simulink model "smm_gait_control"  (R2018b)
settings: configuration reference "Configuration1khz" (kept outside this file)
InitFcn:
  | addpath('./functions/')
  | addpath('./policies/')
  | control_params
values from neighbouring files (symbols this model uses):
  rest = extract_policy_variables('policies/rest.mat')    [control_params.m]
  run_slow = extract_policy_variables('policies/06_run_reduced.mat')    [control_params.m]
  walk_slow = extract_policy_variables('policies/06_walk.mat')    [control_params.m]
undefined symbols (not defined in the file or in its folder): ctrl, Discrete, initial_dx_estimate, initial_dy_estimate, initial_dz_estimate, initial_z_estimate, sample_time, Time
libraries: simulink x42, ctrlSharedLib x7
(part 1 of 5)
settings Model: Creator=wmartin  LastModifiedBy=Will
settings ConfigSetRef: SourceLocation=Base Workspace

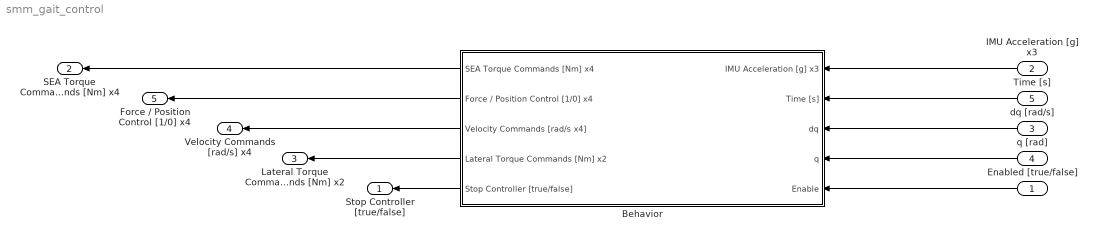
== system smm_gait_control ==
  Enabled [true/false] : Inport  OutDataTypeStr=boolean  PortDimensions=1  SampleTime=sample_time  Interpolate=off
  IMU Acceleration [g] x3 : Inport  Port=2  OutDataTypeStr=double  PortDimensions=3  SampleTime=sample_time  Interpolate=off
  dq [rad/s] : Inport  Port=3  OutDataTypeStr=double  PortDimensions=13  SampleTime=sample_time  Interpolate=off
  q [rad] : Inport  Port=4  OutDataTypeStr=double  PortDimensions=13  SampleTime=sample_time  Interpolate=off
  Time [s] : Inport  Port=5  OutDataTypeStr=double  PortDimensions=1  SampleTime=sample_time  Interpolate=off
  Behavior : Subsystem
  Stop Controller [true/false] : Outport  OutDataTypeStr=boolean  PortDimensions=1  SampleTime=[0.001,0]  OutputWhenDisabled=reset  InitialOutput=[0 0 0 0 0 0]
  SEA Torque Commands [Nm] x4 : Outport  Port=2  OutDataTypeStr=double  PortDimensions=4  SampleTime=[0.001,0]  OutputWhenDisabled=reset  InitialOutput=[0 0 0 0 0 0]
  Lateral Torque Commands [Nm] x2 : Outport  Port=3  OutDataTypeStr=double  PortDimensions=2  SampleTime=[0.001,0]  OutputWhenDisabled=reset  InitialOutput=[0 0 0 0 0 0]
  Velocity Commands [rad/s] x4 : Outport  Port=4  OutDataTypeStr=double  PortDimensions=4  SampleTime=[0.001,0]  OutputWhenDisabled=reset  InitialOutput=[0 0 0 0 0 0]
  Force / Position Control [1/0] x4 : Outport  Port=5  OutDataTypeStr=boolean  PortDimensions=4  SampleTime=[0.001,0]  OutputWhenDisabled=reset  InitialOutput=[0 0 0 0 0 0]
  wires:
  IMU Acceleration [g] x3/1 -> Behavior/1(IMU Acceleration [g] x3)
  dq [rad/s]/1 -> Behavior/3(dq)
  q [rad]/1 -> Behavior/4(q)
  Time [s]/1 -> Behavior/2(Time [s])
  Enabled [true/false]/1 -> Behavior/5(Enable)
  Behavior/5(Stop Controller [true/false]) -> Stop Controller [true/false]/1
  Behavior/1(SEA Torque Commands [Nm] x4) -> SEA Torque Commands [Nm] x4/1
  Behavior/2(Force / Position Control [1/0] x4) -> Force / Position Control [1/0] x4/1
  Behavior/3(Velocity Commands [rad/s x4]) -> Velocity Commands [rad/s] x4/1
  Behavior/4(Lateral Torque Commands [Nm] x2) -> Lateral Torque Commands [Nm] x2/1

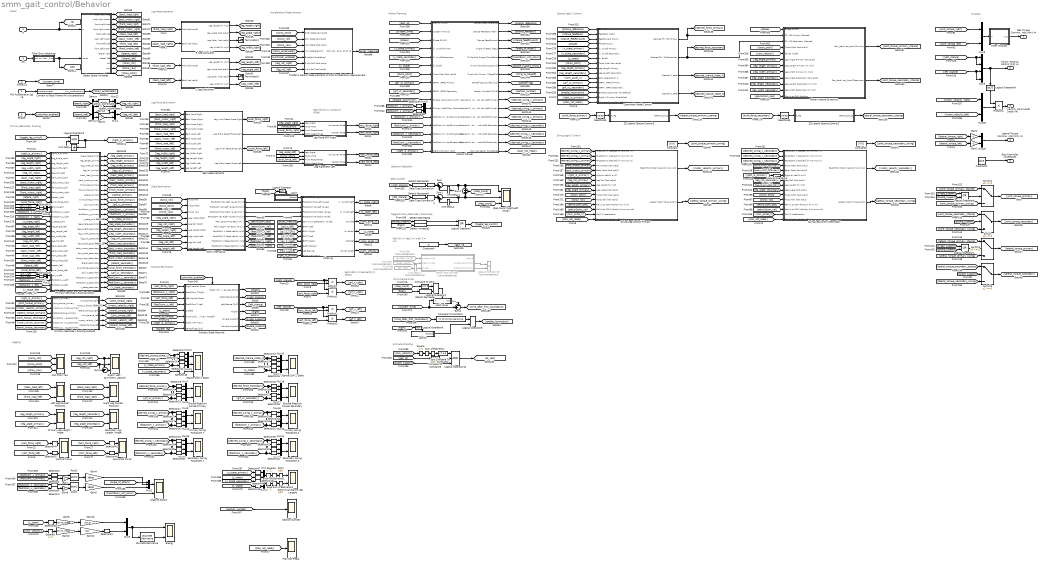
== system smm_gait_control/Behavior ==
  note: Step counter
  note: Gait ID
      | 1 = rest
      | 2 = walk
      | 3 = run
  note: Each GRF is 2 elements
      | [F, dF/dt]
  note: Primary/Secondary Routing
  note: Leg Measurements
  note: Outputs
  note: Inputs
  note: Contact Estimation
  note: Logging
  note: Acceleration Measurement
  note: Swing Leg(s) Control
  note: Leg Force Estimation
  note: Each force is 2 values
      | [F, dF/dt]
  note: State Estimation
  note: Behavior Selection
  note: Toggle Primary/Secondary Role Swap
  note: First stance timer
  note: Activate standing
  note: Motion Planning
  note: Stance Leg(s) Control
  IMU Acceleration [g] x3 : Inport  OutDataTypeStr=double  PortDimensions=3  SampleTime=[0.001,0]
  Time [s] : Inport  Port=2  OutDataTypeStr=double  PortDimensions=1  SampleTime=[0.001,0]
  dq : Inport  Port=3  OutDataTypeStr=double  PortDimensions=13  SampleTime=[0.001,0]
  q : Inport  Port=4  OutDataTypeStr=double  PortDimensions=13  SampleTime=[0.001,0]
  Enable : Inport  Port=5  OutDataTypeStr=boolean  PortDimensions=1  SampleTime=[0.001,0]
  2D Lateral Stance Control2 : MATLAB Function  TreatAsAtomicUnit=on
  2D Lateral Stance Control3 : MATLAB Function  TreatAsAtomicUnit=on
  Angle of Attack : Scope  NumInputPorts=2
  Atan1 : Trigonometry  Operator=atan2
  Atan2 : Trigonometry  Operator=atan2
  Centroidal Model Control : Subsystem
  CoM Kinematics : Subsystem
  Compare To Constant : simulink/Logic and Bit Operations/Compare To Constant  relop=>=  const=ctrl.control_start_time  OutDataTypeStr=boolean
  Compare To Constant2 : simulink/Logic and Bit Operations/Compare To Constant  relop=<=  const=0.5  OutDataTypeStr=boolean
  Compare To Constant3 : simulink/Logic and Bit Operations/Compare To Constant  relop===  const=1  OutDataTypeStr=boolean
  Compare To Zero : simulink/Logic and Bit Operations/Compare To Zero  relop===  OutDataTypeStr=boolean
  Constant : Constant  Value=[0 0]
  Constant2 : Constant  Value=false
  Constant4 : Constant  Value=3
  Constant5 : Constant  Value=[0 0]
  Contact State Machine : Subsystem
  Convert to Body Frame IMU Accelerations : MATLAB Function  TreatAsAtomicUnit=on
  Data Type Conversion : DataTypeConversion  OutDataTypeStr=double
  Data Type Conversion1 : DataTypeConversion  OutDataTypeStr=double
  Demux : Demux  Outputs=2
  Demux1 : Demux  Outputs=2
  Detect Decrease : simulink/Logic and Bit Operations/Detect Decrease  vinit=0.0  OutDataTypeStr=boolean
  Detect Decrease2 : simulink/Logic and Bit Operations/Detect Decrease  vinit=0  OutDataTypeStr=boolean
  Detect Decrease3 : simulink/Logic and Bit Operations/Detect Decrease  vinit=0.0  OutDataTypeStr=boolean
  Detect Decrease4 : simulink/Logic and Bit Operations/Detect Decrease  vinit=0  OutDataTypeStr=boolean
  Detect Increase2 : simulink/Logic and Bit Operations/Detect Increase  vinit=1  OutDataTypeStr=boolean
  Discrete Derivative : simulink/Discrete/Discrete Derivative  gainval=1.0  ICPrevScaledInput=0.0  OutMin=[]  OutMax=[]  OutDataType=fixdt(1, 16)  OutScaling=2^-10  DoSatur=off
  Energy : Scope  NumInputPorts=2
  Filter Gyro Velocities : Subsystem
  Filter Torques : Subsystem
  Filtering : Subsystem
  From258 : From  Commented=on  GotoTag=system_time
  From259 : From  Commented=on  GotoTag=step_count
  From260 : From  Commented=on  GotoTag=at_rest
  Gain{,1..3,6,12} (6 alike) : Gain  Gain=-1
  Gain10 : Gain  Gain=ctrl.m_total
  Gain11 : Gain  Gain=0.5
  Gain13 : Gain  Gain=ctrl.g
  Gain4 : Gain  Gain=180/pi
  Gain5 : Gain  Gain=180/pi
  Gain9 : Gain  Gain=ctrl.m_total
  Ground Reaction Forces Primary : Scope  NumInputPorts=2
  Ground Reaction Forces Secondary : Scope  NumInputPorts=2
  Hold Value : Subsystem  TreatAsAtomicUnit=on
  Horizontal Force : Scope  NumInputPorts=2
  L Leg Calculator : Subsystem
  Latch : Subsystem  TreatAsAtomicUnit=on
  Latch2 : Subsystem  TreatAsAtomicUnit=on
  Left Leg Fourbar Positions : Scope  NumInputPorts=2
  Leg Plane GRF Left : Subsystem
  Leg Plane GRF Right : Subsystem
  Logical Operator{,5..6,9} (4 alike) : Logic  Operator=NOT  AllPortsSameDT=off  OutDataTypeStr=boolean
  Logical Operator1 : Logic  Operator=OR  AllPortsSameDT=off  OutDataTypeStr=boolean
  Logical Operator10 : Logic  Inputs=3  AllPortsSameDT=off  OutDataTypeStr=boolean
  Logical Operator15 : Logic  Commented=on  Operator=OR  AllPortsSameDT=off  OutDataTypeStr=boolean
  Logical Operator2 : Logic  AllPortsSameDT=off  OutDataTypeStr=boolean
  Logical Operator3 : Logic  Operator=XOR  AllPortsSameDT=off  OutDataTypeStr=boolean
  Logical Operator4 : Logic  Operator=OR  AllPortsSameDT=off  OutDataTypeStr=boolean
  Logical Operator7 : Logic  Operator=OR  AllPortsSameDT=off  OutDataTypeStr=boolean
  Logical Operator8 : Logic  AllPortsSameDT=off  OutDataTypeStr=boolean
  Motion Planner : Subsystem
  Mux{,1,4..26,28..29} (27 alike) : Mux  Inputs=2
  Mux2 : Mux  Inputs=3
  Mux3 : Mux
  Plan Not Ready : Scope
  Planar Inverse Dynamics : Subsystem
  Primary Leg Length / Angle : Scope  NumInputPorts=2
  Primary Swing Foot2CoM X : Scope  NumInputPorts=2
  Primary Swing Foot2CoM Z : Scope  NumInputPorts=2
  Primary-Secondary Routing Inputs : MATLAB Function  TreatAsAtomicUnit=on
  Primary-Secondary Routing Outputs : MATLAB Function  TreatAsAtomicUnit=on
  Product{,1..4} (5 alike) : Product
  R Leg Calculator : Subsystem
  Right / Left / Symmetry Leg Roll : Scope  NumInputPorts=3
  Right Leg Fourbar Positions : Scope  NumInputPorts=2
  Roll Pitch Yaw : Scope  NumInputPorts=3
  SEA Measurements : Subsystem
  Secondary Leg Length / Angle : Scope  NumInputPorts=2
  Secondary Swing Foot2CoM X : Scope  NumInputPorts=2
  Secondary Swing Foot2CoM Z : Scope  NumInputPorts=2
  Section Number : Scope
  Select Gait Number : MATLAB Function  Commented=on  TreatAsAtomicUnit=on
  Select State Variables : Subsystem
  Selector{10,12,15..16,21..23,28,30,32,38,40} (12 alike) : Selector  InputPortWidth=2  IndexOptions=Index vector (dialog)  Indices=[2]  OutputSizes=1
  Selector{11,18,34,36} (4 alike) : Selector  InputPortWidth=3  IndexOptions=Index vector (dialog)  Indices=[1]  OutputSizes=1
  Selector{2..9,13..14,20,24..27,29,31,33,39,41..52,55..58} (35 alike) : Selector  InputPortWidth=2  IndexOptions=Index vector (dialog)  Indices=[1]  OutputSizes=1
  Selector{17,19,35,37} (4 alike) : Selector  InputPortWidth=3  IndexOptions=Index vector (dialog)  Indices=[2]  OutputSizes=1
  Sqrt : Sqrt  SaturateOnIntegerOverflow=on
  Sqrt1 : Sqrt  SaturateOnIntegerOverflow=on
  Sqrt2 : Sqrt  SaturateOnIntegerOverflow=on
  Square{,1..3} (4 alike) : Math  Operator=square  SaturateOnIntegerOverflow=on
  Stance CoM X State : Scope  NumInputPorts=3
  Stance CoM Z State : Scope  NumInputPorts=2
  Step Count (Right/Left/Total) : Scope  NumInputPorts=3
  Sum : Sum  Inputs=|++
  Sum of Elements : Sum  Inputs=+
  Sum of Elements1 : Sum  Inputs=+
  Sum of Elements2 : Sum  Inputs=+
  Sum1 : Sum  Inputs=|++
  Sum2 : Sum  Inputs=+|+
  Sum3 : Sum  Inputs=-+|
  Sum4 : Sum  Inputs=-+|
  Swing Leg Control Primary : Subsystem
  Swing Leg Control Secondary : Subsystem
  Switch{,1..3} (4 alike) : Switch  Criteria=u2 ~= 0  Threshold=2
  Terminator2 : Terminator
  Terminator3 : Terminator
  Tranform Sensor Measurements to CoM Acceleration Measurement : Subsystem
  Unit Delay : UnitDelay  InitialCondition=ctrl.initial_leg_selection  SampleTime=sample_time
  Unit Delay1 : UnitDelay  SampleTime=-1
  Unit Delay2 : UnitDelay  SampleTime=-1
  Unit Delay4 : UnitDelay  Commented=on  SampleTime=-1
  Vertical Force : Scope  NumInputPorts=2
  Virtual Stance Leg Lengths : Scope  NumInputPorts=2
  lateral_coordinates : Fcn  Expr=pi/2-u
  lateral_coordinates1 : Fcn  Expr=pi/2-u
  SEA Torque Commands [Nm] x4 : Outport  OutDataTypeStr=double  PortDimensions=4  SampleTime=[0.001,0]  OutputWhenDisabled=reset  InitialOutput=[0 0 0 0]
  Force / Position Control [1/0] x4 : Outport  Port=2  OutDataTypeStr=boolean  PortDimensions=4  SampleTime=[0.001,0]  OutputWhenDisabled=reset  InitialOutput=[0 0 0 0]
  Velocity Commands [rad/s x4] : Outport  Port=3  OutDataTypeStr=double  PortDimensions=4  SampleTime=[0.001,0]  OutputWhenDisabled=reset  InitialOutput=[0 0 0 0]
  Lateral Torque Commands [Nm] x2 : Outport  Port=4  OutDataTypeStr=double  PortDimensions=2  SampleTime=[0.001,0]  OutputWhenDisabled=reset  InitialOutput=[0 0]
  Stop Controller [true/false] : Outport  Port=5  OutDataTypeStr=boolean  PortDimensions=1  SampleTime=[0.001,0]  OutputWhenDisabled=reset  InitialOutput=0
  wires:
  [leg_roll_right] -> Sum3/1, Right / Left / Symmetry Leg Roll/1
  [torso_pitch] -> Roll Pitch Yaw/2
  [leg_roll_left] -> Sum3/2, Right / Left / Symmetry Leg Roll/2
  Sum3/1 -> Right / Left / Symmetry Leg Roll/3
  [leg_length_primary] -> Primary Leg Length / Angle/1
  [leg_angle_primary] -> Primary Leg Length / Angle/2
  [leg_length_secondary] -> Secondary Leg Length / Angle/1
  [leg_angle_secondary] -> Secondary Leg Length / Angle/2
  [torso_roll] -> Roll Pitch Yaw/1
  [torso_yaw] -> Roll Pitch Yaw/3
  Time [s]/1 -> [system_time]
  Demux/2 -> Gain12/1
  lateral_coordinates/1 -> Mux22/1
  [back_load_left] -> Left Leg Fourbar Positions/1
  Gain12/1 -> Mux22/2
  [back_load_right] -> Right Leg Fourbar Positions/1
  Mux22/1 -> [leg_roll_right]
  Demux/1 -> lateral_coordinates/1
  [front_load_right] -> Right Leg Fourbar Positions/2
  [front_load_left] -> Left Leg Fourbar Positions/2
  [lateral_torque_right] -> Gain2/1
  L Leg Calculator/4(Leg Width [m m/s]) -> [leg_width_left]
  q/1 -> [q], Select State Variables/1(q)
  R Leg Calculator/4(Leg Width [m m/s]) -> [leg_width_right]
  L Leg Calculator/3(Leg Splay [rad rad/s]) -> Terminator3/1
  L Leg Calculator/2(Leg Angle [rad rad/s]) -> [leg_angle_left]
  L Leg Calculator/1("Leg Length [m m/s] ") -> [leg_length_left]
  R Leg Calculator/3(Leg Splay [rad rad/s]) -> Terminator2/1
  [lateral_torque_left] -> Gain1/1
  [back_load_right] -> R Leg Calculator/2(Back [rad rad/s])
  [front_load_right] -> R Leg Calculator/1(Front [rad rad/s])
  R Leg Calculator/2(Leg Angle [rad rad/s]) -> [leg_angle_right]
  R Leg Calculator/1("Leg Length [m m/s] ") -> [leg_length_right]
  [joint_torque_right] -> Mux8/1
  [joint_torque_left] -> Mux8/2
  [left_stance] -> Mux3/3, Mux3/4
  [right_stance] -> Mux3/2, Mux3/1
  Mux3/1 -> Logical Operator9/1, Force / Position Control [1/0] x4/1
  Gain2/1 -> Mux25/1
  Mux25/1 -> Lateral Torque Commands [Nm] x2/1
  Gain1/1 -> Mux25/2
  [torso_pitch] -> Tranform Sensor Measurements to CoM Acceleration Measurement/1(Pitch State [rad rad/s])
  [torso_accelmeter] -> Tranform Sensor Measurements to CoM Acceleration Measurement/4(Imu Accelerations)
  [controller_enabled] -> Tranform Sensor Measurements to CoM Acceleration Measurement/5(Enabled [true/false])
  Tranform Sensor Measurements to CoM Acceleration Measurement/1(CoM Acceleration [m/s] x3) -> [accel_measure]
  [leg_roll_right] -> Tranform Sensor Measurements to CoM Acceleration Measurement/6(R Hip Roll [rad rad/s])
  [leg_roll_left] -> Tranform Sensor Measurements to CoM Acceleration Measurement/7(L Hip Roll [rad rad/s])
  [torso_roll] -> Tranform Sensor Measurements to CoM Acceleration Measurement/2(Roll State [rad rad/s])
  [torso_yaw] -> Tranform Sensor Measurements to CoM Acceleration Measurement/3(Yaw State [rad rad/s])
  Constant2/1 -> Stop Controller [true/false]/1
  dq/1 -> Filter Gyro Velocities/1(raw dq)
  Select State Variables/1(back right load) -> [back_load_right]
  Select State Variables/2(back right motor) -> [back_motor_right]
  Select State Variables/3(front right load) -> [front_load_right]
  Select State Variables/4(front right motor) -> [front_motor_right]
  Select State Variables/5(back left load) -> [back_load_left]
  Select State Variables/6(back left motor) -> [back_motor_left]
  Select State Variables/7(front left load) -> [front_load_left]
  Select State Variables/8(front left motor) -> [front_motor_left]
  Select State Variables/13(pitch) -> [torso_pitch]
  Select State Variables/12(yaw) -> [torso_yaw]
  Select State Variables/11(roll) -> [torso_roll]
  Select State Variables/10(lateral left) -> [lateral_left]
  Select State Variables/9(lateral right) -> [lateral_right]
  Logical Operator3/1 -> [right_is_primary], Unit Delay/1
  [toggle_leg_switch] -> Logical Operator3/1
  Unit Delay/1 -> Logical Operator3/2
  [front_load_left] -> L Leg Calculator/1(Front [rad rad/s])
  [back_load_left] -> L Leg Calculator/2(Back [rad rad/s])
  [lateral_right] -> Demux/1
  [lateral_left] -> Demux1/1
  Demux1/1 -> lateral_coordinates1/1
  Mux1/1 -> [leg_roll_left]
  Gain3/1 -> Mux1/2
  lateral_coordinates1/1 -> Mux1/1
  Demux1/2 -> Gain3/1
  Primary-Secondary Routing Inputs/1(leg_angle_primary) -> [leg_angle_primary]
  [leg_angle_right] -> Primary-Secondary Routing Inputs/2(leg_angle_right)
  [leg_length_right] -> Primary-Secondary Routing Inputs/3(leg_length_right)
  [leg_width_right] -> Primary-Secondary Routing Inputs/4(leg_width_right)
  [leg_roll_right] -> Primary-Secondary Routing Inputs/5(leg_roll_right)
  [back_load_right] -> Primary-Secondary Routing Inputs/6(back_load_right)
  [back_motor_right] -> Primary-Secondary Routing Inputs/7(back_motor_right)
  [front_load_right] -> Primary-Secondary Routing Inputs/8(front_load_right)
  [front_motor_right] -> Primary-Secondary Routing Inputs/9(front_motor_right)
  [lateral_right] -> Primary-Secondary Routing Inputs/10(lateral_right)
  [leg_angle_left] -> Primary-Secondary Routing Inputs/16(leg_angle_left)
  [leg_length_left] -> Primary-Secondary Routing Inputs/17(leg_length_left)
  [leg_width_left] -> Primary-Secondary Routing Inputs/18(leg_width_left)
  [leg_roll_left] -> Primary-Secondary Routing Inputs/19(leg_roll_left)
  [back_load_left] -> Primary-Secondary Routing Inputs/20(back_load_left)
  [back_motor_left] -> Primary-Secondary Routing Inputs/21(back_motor_left)
  [front_load_left] -> Primary-Secondary Routing Inputs/22(front_load_left)
  [front_motor_left] -> Primary-Secondary Routing Inputs/23(front_motor_left)
  [lateral_left] -> Primary-Secondary Routing Inputs/24(lateral_left)
  Primary-Secondary Routing Inputs/23(lateral_secondary) -> [lateral_secondary]
  Primary-Secondary Routing Inputs/22(front_motor_secondary) -> [front_motor_secondary]
  Primary-Secondary Routing Inputs/21(front_load_secondary) -> [front_load_secondary]
  Primary-Secondary Routing Inputs/20(back_motor_secondary) -> [back_motor_secondary]
  Primary-Secondary Routing Inputs/19(back_load_secondary) -> [back_load_secondary]
  Primary-Secondary Routing Inputs/18(leg_roll_secondary) -> [leg_roll_secondary]
  Primary-Secondary Routing Inputs/17(leg_width_secondary) -> [leg_width_secondary]
  Primary-Secondary Routing Inputs/16(leg_length_secondary) -> [leg_length_secondary]
  Primary-Secondary Routing Inputs/15(leg_angle_secondary) -> [leg_angle_secondary]
  Primary-Secondary Routing Inputs/9(lateral_primary) -> [lateral_primary]
  Primary-Secondary Routing Inputs/8(front_motor_primary) -> [front_motor_primary]
  Primary-Secondary Routing Inputs/7(front_load_primary) -> [front_load_primary]
  Primary-Secondary Routing Inputs/6(back_motor_primary) -> [back_motor_primary]
  Primary-Secondary Routing Inputs/5(back_load_primary) -> [back_load_primary]
  Primary-Secondary Routing Inputs/4(leg_roll_primary) -> [leg_roll_primary]
  Primary-Secondary Routing Inputs/3(leg_width_primary) -> [leg_width_primary]
  Primary-Secondary Routing Inputs/2(leg_length_primary) -> [leg_length_primary]
  Enable/1 -> [controller_enabled]
  Convert to Body Frame IMU Accelerations/1(imu_accelerations) -> [torso_accelmeter]
  IMU Acceleration [g] x3/1 -> Convert to Body Frame IMU Accelerations/1(accelerometer)
  [vert_force_right] -> Contact State Machine/1(Right Vertical Force)
  [vert_force_left] -> Contact State Machine/3(Left Vertical Force)
  [back_load_right] -> SEA Measurements/1(Back Load Right)
  [back_motor_right] -> SEA Measurements/2(Back Motor Right)
  [front_load_right] -> SEA Measurements/3(Front Load Right)
  [front_motor_right] -> SEA Measurements/4(Front Motor Right)
  [back_load_left] -> SEA Measurements/5(Back Load Left)
  [back_motor_left] -> SEA Measurements/6(Back Motor Left)
  [front_load_left] -> SEA Measurements/7(Front Load Left)
  [front_motor_left] -> SEA Measurements/8(Front Motor Left)
  [leg_width_right] -> SEA Measurements/9(Leg Width Right)
  [leg_length_left] -> SEA Measurements/12(Leg Length Left)
  [leg_length_right] -> SEA Measurements/10(Leg Length Right)
  [leg_width_left] -> SEA Measurements/11(Leg Width Left)
  SEA Measurements/2(Leg Ortho React Force Right) -> Leg Plane GRF Right/4(Ortho React Force)
  [torso_pitch] -> Leg Plane GRF Right/2(Torso Pitch)
  [leg_angle_right] -> Leg Plane GRF Right/1(Leg Angle)
  [leg_angle_left] -> Leg Plane GRF Left/1(Leg Angle)
  [torso_pitch] -> Leg Plane GRF Left/2(Torso Pitch)
  Leg Plane GRF Right/2(Vertical Force) -> [vert_force_right]
  [vert_force_right] -> Selector44/1
  [vert_force_left] -> Selector52/1
  [horz_force_right] -> Selector42/1
  [horz_force_left] -> Selector43/1
  [torso_pitch] -> CoM Kinematics/2(Torso Pitch)
  [torso_roll] -> CoM Kinematics/1(Torso Roll)
  [torso_yaw] -> CoM Kinematics/3(Torso Yaw)
  [leg_length_left] -> CoM Kinematics/9(Leg Length Left)
  [leg_length_right] -> CoM Kinematics/6(Leg Length Right)
  [leg_angle_right] -> CoM Kinematics/4(Leg Angle Right)
  [leg_angle_left] -> CoM Kinematics/7(Leg Angle Left)
  [leg_roll_left] -> CoM Kinematics/8(Leg Roll Left)
  [leg_roll_right] -> CoM Kinematics/5(Leg Roll Right)
  Contact State Machine/2(Right Stance [1/0]) -> [right_stance]
  Contact State Machine/3(Left Stance [1/0]) -> [left_stance]
  [horz_force_right] -> Product/2
  [vert_force_right] -> Product1/2
  [right_stance] -> Product1/1, Product/1
  [vert_force_left] -> Product3/2
  [horz_force_left] -> Product2/2
  [left_stance] -> Product3/1, Product2/1
  Product/1 -> [grf_x_right]
  Product1/1 -> [grf_z_right]
  Product2/1 -> [grf_x_left]
  Product3/1 -> [grf_z_left]
  CoM Kinematics/1(Foot2CoM Pos Left Yawed [m] x3) -> Filtering/2(Foot2CoM Pos Left Yawed)
  CoM Kinematics/2(Foot2CoM Vel Left Yawed [m/s] x3) -> Filtering/3(Foot2CoM Vel Left Yawed)
  CoM Kinematics/3(Foot2CoM Pos Right Yawed [m] x3) -> Filtering/4(Foot2CoM Pos Right Yawed)
  CoM Kinematics/4(Foot2CoM Vel Right Yawed [m/s] x3) -> Filtering/5(Foot2CoM Vel Right Yawed)
  [accel_measure] -> Filtering/6(CoM XYZ Acceleration Yawed)
  [grf_x_left] -> Filtering/7(GRF X Left)
  [grf_x_right] -> Filtering/8(GRF X Right)
  [grf_z_left] -> Filtering/9(GRF Z Left)
  [grf_z_right] -> Filtering/10(GRF Z Right)
  [right_stance] -> Filtering/11(Right Stance?)
  [left_stance] -> Filtering/12(Left Stance?)
  [right_is_primary] -> Filtering/13(Right Is Primary?)
  Filtering/1("[x, dx/dt] Right") -> [x_state_right]
  Filtering/2("[x, dx/dt] Left") -> [x_state_left]
  Filtering/3(ddx/ddt) -> [com_accel_x]
  Filtering/4("[z, dz/dt]") -> [z_state]
  Filtering/5(ddz/ddt) -> [com_accel_z]
  [flight] -> Logical Operator/1
  Logical Operator/1 -> Latch/Enable
  Contact State Machine/4(Flight?) -> [flight]
  Contact State Machine/1(Flight / Single / Double [0/1/2]) -> [phase]
  Contact State Machine/5(Single Support?) -> [single_support]
  Contact State Machine/6(Double Support?) -> [double_support]
  Latch/1(latched) -> Filtering/1(Enable Filtering)
  CoM Kinematics/5(Pelvis2CoM Pos Body [m] x3) -> [pelvis2com_pos]
  CoM Kinematics/6(Pelvis2CoM Vel Body [m/s] x3) -> [pelvis2com_vel]
  Primary-Secondary Routing Outputs/1(joint_torque_right) -> [joint_torque_right]
  Primary-Secondary Routing Outputs/2(motor_velocity_right) -> [motor_velocity_right]
  Primary-Secondary Routing Outputs/6(lateral_torque_left) -> [lateral_torque_left]
  Primary-Secondary Routing Outputs/5(motor_velocity_left) -> [motor_velocity_left]
  Primary-Secondary Routing Outputs/4(joint_torque_left) -> [joint_torque_left]
  Primary-Secondary Routing Outputs/3(lateral_torque_right) -> [lateral_torque_right]
  [joint_torque_secondary] -> Primary-Secondary Routing Outputs/5(joint_torque_secondary)
  [motor_velocity_secondary] -> Primary-Secondary Routing Outputs/6(motor_velocity_secondary)
  [lateral_torque_secondary] -> Primary-Secondary Routing Outputs/7(lateral_torque_secondary)
  [lateral_torque_primary] -> Primary-Secondary Routing Outputs/4(lateral_torque_primary)
  [motor_velocity_primary] -> Primary-Secondary Routing Outputs/3(motor_velocity_primary)
  [joint_torque_primary] -> Primary-Secondary Routing Outputs/2(joint_torque_primary)
  [right_is_primary] -> Primary-Secondary Routing Inputs/1(right_is_primary)
  [right_is_primary] -> Primary-Secondary Routing Outputs/1(right_is_primary)
  Filtering/6("[dx/dt, dz/dt]") -> [com_velocity]
  [desired_swing_x_secondary] -> Swing Leg Control Secondary/1(Foot2CoM X Desired [m m/s m/s^2])
  [desired_swing_z_secondary] -> Swing Leg Control Secondary/3(Foot2CoM Z Desired [m m/s m/s^2])
  [pelvis2com_vel] -> Swing Leg Control Secondary/13(Pelvis to COM Velocity [m/s m/s m/s])
  [pelvis2com_pos] -> Swing Leg Control Secondary/12(Pelvis to COM Position [m m m])
  [torso_pitch] -> Swing Leg Control Secondary/10(Torso Pitch [rad rad/s])
  [torso_roll] -> Swing Leg Control Secondary/11(Torso Roll [rad rad/s])
  [right_is_primary] -> Logical Operator5/1
  [back_motor_secondary] -> Swing Leg Control Secondary/5(Back Motor [rad rad/s])
  [front_motor_secondary] -> Swing Leg Control Secondary/4(Front Motor [rad rad/s])
  [leg_roll_secondary] -> Swing Leg Control Secondary/7(Leg Roll [rad rad/s])
  [leg_length_secondary] -> Swing Leg Control Secondary/8(Leg Length [m m/s])
  [leg_angle_secondary] -> Swing Leg Control Secondary/9(Leg Angle [rad rad/s])
  Switch/1 -> [joint_torque_secondary]
  [double_support] -> Switch/2
  [desired_swing_y_secondary] -> Swing Leg Control Secondary/2(Foot2CoM Y Desired [m m/s m/s^2])
  SEA Measurements/1(Leg Axial React Force Right) -> [axial_force_right]
  SEA Measurements/3(Leg Axial React Force Left) -> [axial_force_left]
  [axial_force_right] -> Leg Plane GRF Right/3(Axial React Force)
  [axial_force_left] -> Leg Plane GRF Left/3(Axial React Force)
  [axial_force_right] -> Primary-Secondary Routing Inputs/11(axial_force_right)
  [axial_force_left] -> Primary-Secondary Routing Inputs/25(axial_force_left)
  Primary-Secondary Routing Inputs/24(axial_force_secondary) -> [axial_force_secondary]
  Primary-Secondary Routing Inputs/10(axial_force_primary) -> [axial_force_primary]
  [single_support] -> Logical Operator1/1
  [double_support] -> Logical Operator1/2
  Logical Operator1/1 -> Switch2/2
  Switch2/1 -> [lateral_torque_primary]
  [joint_torque_secondary_stance] -> Switch/1
  Swing Leg Control Secondary/1(Back/Front Motor Velocity [m/s m/s]) -> [motor_velocity_secondary]
  [joint_torque_secondary_swing] -> Switch/3
  [lateral_torque_primary_stance] -> Switch2/1
  [lateral_torque_primary_swing] -> Switch2/3
  Switch3/1 -> [lateral_torque_secondary]
  [double_support] -> Switch3/2
  Swing Leg Control Secondary/2(Lateral Motor Torque [Nm]) -> [lateral_torque_secondary_swing]
  [lateral_torque_secondary_stance] -> Switch3/1
  [lateral_torque_secondary_swing] -> Switch3/3
  [joint_torque_primary_swing] -> Switch1/3
  [joint_torque_primary_stance] -> Switch1/1
  Logical Operator4/1 -> Switch1/2
  Switch1/1 -> [joint_torque_primary]
  [double_support] -> Logical Operator4/2
  [single_support] -> Logical Operator4/1
  [com_accel_z] -> Swing Leg Control Secondary/14(CoM Z Acceleration)
  [com_accel_z] -> Swing Leg Control Primary/14(CoM Z Acceleration)
  [desired_swing_y_primary] -> Swing Leg Control Primary/2(Foot2CoM Y Desired [m m/s m/s^2])
  [leg_angle_primary] -> Swing Leg Control Primary/9(Leg Angle [rad rad/s])
  [leg_length_primary] -> Swing Leg Control Primary/8(Leg Length [m m/s])
  [leg_roll_primary] -> Swing Leg Control Primary/7(Leg Roll [rad rad/s])
  [front_motor_primary] -> Swing Leg Control Primary/4(Front Motor [rad rad/s])
  [back_motor_primary] -> Swing Leg Control Primary/5(Back Motor [rad rad/s])
  [right_is_primary] -> Swing Leg Control Primary/6(Right or Left [1 or 0])
  [torso_roll] -> Swing Leg Control Primary/11(Torso Roll [rad rad/s])
  [torso_pitch] -> Swing Leg Control Primary/10(Torso Pitch [rad rad/s])
  [pelvis2com_pos] -> Swing Leg Control Primary/12(Pelvis to COM Position [m m m])
  [pelvis2com_vel] -> Swing Leg Control Primary/13(Pelvis to COM Velocity [m/s m/s m/s])
  [desired_swing_z_primary] -> Swing Leg Control Primary/3(Foot2CoM Z Desired [m m/s m/s^2])
  [desired_swing_x_primary] -> Swing Leg Control Primary/1(Foot2CoM X Desired [m m/s m/s^2])
  Swing Leg Control Primary/1(Back/Front Motor Velocity [m/s m/s]) -> [motor_velocity_primary]
  Swing Leg Control Primary/2(Lateral Motor Torque [Nm]) -> [lateral_torque_primary_swing]
  Logical Operator5/1 -> Swing Leg Control Secondary/6(Right or Left [1 or 0])
  [x_state_right] -> Primary-Secondary Routing Inputs/15(x_state_right)
  [x_state_left] -> Primary-Secondary Routing Inputs/29(x_state_left)
  Primary-Secondary Routing Inputs/14(x_state_primary) -> [x_state_primary]
  Primary-Secondary Routing Inputs/28(x_state_secondary) -> [x_state_secondary]
  Leg Plane GRF Right/1(Horizontal Force) -> [horz_force_right]
  Leg Plane GRF Left/1(Horizontal Force) -> [horz_force_left]
  Leg Plane GRF Left/2(Vertical Force) -> [vert_force_left]
  SEA Measurements/4(Leg Ortho React Force Left) -> Leg Plane GRF Left/4(Ortho React Force)
  [double_support] -> Detect Decrease3/1
  [flight] -> Detect Increase2/1
  [desired_stance_state_z] -> Selector15/1, Selector13/1
  Selector12/1 -> Mux13/2
  Mux11/1 -> Stance CoM Z State/2
  Selector13/1 -> Mux10/1
  Mux10/1 -> Stance CoM Z State/1
  Selector6/1 -> Mux12/1
  Selector14/1 -> Mux10/2
  [z_state] -> Selector14/1, Selector16/1
  [x_state_primary] -> Selector7/1, Selector12/1
  Selector16/1 -> Mux11/2
  Mux13/1 -> Stance CoM X State/2
  Selector15/1 -> Mux11/1
  Selector7/1 -> Mux12/2
  Selector10/1 -> Mux13/1
  Mux12/1 -> Stance CoM X State/1
  [desired_stance_state_x] -> Selector6/1, Selector10/1
  Mux9/1 -> Primary Swing Foot2CoM X/1
  Mux14/1 -> Primary Swing Foot2CoM X/2
  [desired_swing_x_primary] -> Selector17/1, Selector11/1
  Selector11/1 -> Mux9/1
  Selector17/1 -> Mux14/1
  Selector19/1 -> Mux15/1
  Selector18/1 -> Mux16/1
  [desired_swing_z_primary] -> Selector18/1, Selector19/1
  Mux15/1 -> Primary Swing Foot2CoM Z/2
  Mux16/1 -> Primary Swing Foot2CoM Z/1
  CoM Kinematics/7(Foot2CoM X State Left [m m/s]) -> [foot2com_x_left]
  CoM Kinematics/8(Foot2CoM Z State Left [m m/s]) -> [foot2com_z_left]
  CoM Kinematics/9(Foot2CoM X State Right [m m/s]) -> [foot2com_x_right]
  CoM Kinematics/10(Foot2CoM Z State Right [m m/s]) -> [foot2com_z_right]
  Mux6/1 -> Ground Reaction Forces Primary/2
  Mux7/1 -> Ground Reaction Forces Primary/1
  [desired_force_primary] -> Selector22/1, Selector8/1
  Selector8/1 -> Mux7/1
  Selector22/1 -> Mux6/1
  Selector21/1 -> Mux17/1
  [desired_force_secondary] -> Selector21/1, Selector20/1
  Selector20/1 -> Mux18/1
  Mux18/1 -> Ground Reaction Forces Secondary/1
  Mux17/1 -> Ground Reaction Forces Secondary/2
  [grf_z_right] -> Selector24/1
  [grf_x_right] -> Selector9/1
  [foot2com_x_right] -> Primary-Secondary Routing Inputs/13(foot2com_x_right)
  [foot2com_z_right] -> Primary-Secondary Routing Inputs/14(foot2com_z_right)
  [foot2com_x_left] -> Primary-Secondary Routing Inputs/27(foot2com_x_left)
  [foot2com_z_left] -> Primary-Secondary Routing Inputs/28(foot2com_z_left)
  Selector9/1 -> Mux19/1
  Selector24/1 -> Mux19/2
  Mux19/1 -> Primary-Secondary Routing Inputs/12(grf_xz_right)
  Selector26/1 -> Mux20/2
  Selector27/1 -> Mux20/1
  [grf_x_left] -> Selector27/1
  Mux20/1 -> Primary-Secondary Routing Inputs/26(grf_xz_left)
  [grf_z_left] -> Selector26/1
  Primary-Secondary Routing Inputs/12(foot2com_x_primary) -> [foot2com_x_primary]
  Primary-Secondary Routing Inputs/13(foot2com_z_primary) -> [foot2com_z_primary]
  Primary-Secondary Routing Inputs/11(grf_xz_primary) -> [grf_xz_primary]
  Primary-Secondary Routing Inputs/25(grf_xz_secondary) -> [grf_xz_secondary]
  Primary-Secondary Routing Inputs/26(foot2com_x_secondary) -> [foot2com_x_secondary]
  Primary-Secondary Routing Inputs/27(foot2com_z_secondary) -> [foot2com_z_secondary]
  Selector25/1 -> Mux7/2
  Selector23/1 -> Mux6/2
  [grf_xz_primary] -> Selector25/1, Selector23/1
  Selector29/1 -> Mux18/2
  Selector28/1 -> Mux17/2
  [grf_xz_secondary] -> Selector28/1, Selector29/1
  Selector31/1 -> Mux9/2
  Selector30/1 -> Mux14/2
  [foot2com_x_primary] -> Selector30/1, Selector31/1
  Selector33/1 -> Mux16/2
  Selector32/1 -> Mux15/2
  [foot2com_z_primary] -> Selector33/1, Selector32/1
  [foot2com_z_secondary] -> Selector40/1, Selector41/1
  Selector40/1 -> Mux23/2
  Selector41/1 -> Mux24/2
  [foot2com_x_secondary] -> Selector39/1, Selector38/1
  Selector38/1 -> Mux21/2
  Selector39/1 -> Mux26/2
  Mux24/1 -> Secondary Swing Foot2CoM Z/1
  Mux23/1 -> Secondary Swing Foot2CoM Z/2
  [desired_swing_z_secondary] -> Selector37/1, Selector36/1
  Selector36/1 -> Mux24/1
  Selector37/1 -> Mux23/1
  Selector35/1 -> Mux21/1
  Selector34/1 -> Mux26/1
  [desired_swing_x_secondary] -> Selector34/1, Selector35/1
  Mux21/1 -> Secondary Swing Foot2CoM X/2
  Mux26/1 -> Secondary Swing Foot2CoM X/1
  [angle_of_attack] -> Mux2/1
  [touchdown_will_occur] -> Angle of Attack/2
  Logical Operator8/1 -> [enable_locomotion]
  Mux2/1 -> Angle of Attack/1
  Atan2/1 -> Gain4/1
  [foot2com_z_primary] -> Selector3/1
  [foot2com_x_primary] -> Selector2/1
  Selector2/1 -> Gain/1
  Gain4/1 -> Mux2/2
  Selector3/1 -> Atan2/1
  Gain/1 -> Atan2/2
  Gain5/1 -> Mux2/3
  Gain6/1 -> Atan1/2
  Selector5/1 -> Atan1/1
  Selector4/1 -> Gain6/1
  Atan1/1 -> Gain5/1
  [foot2com_x_secondary] -> Selector4/1
  [foot2com_z_secondary] -> Selector5/1
  [flight] -> Detect Decrease/1
  Square/1 -> Sum of Elements/1
  Sum of Elements/1 -> Sqrt/1
  Logical Operator7/1 -> [toggle_leg_switch]
  [com_velocity] -> Square/1
  Sqrt/1 -> Compare To Constant2/1
  Compare To Constant2/1 -> Logical Operator10/1
  [z_state] -> Contact State Machine/5(Z State)
  [foot2com_z_left] -> Contact State Machine/4(Foot2Com Z Left)
  [foot2com_z_right] -> Contact State Machine/2(Foot2Com Z Right)
  Detect Decrease3/1 -> Logical Operator7/1
  Detect Increase2/1 -> Logical Operator7/2
  [gait_id] -> Compare To Constant3/1
  Compare To Constant3/1 -> Logical Operator10/2
  [x_state_secondary] -> Selector45/1
  Selector45/1 -> Stance CoM X State/3
  Sum of Elements1/1 -> Sqrt1/1
  Square1/1 -> Sum of Elements1/1
  [x_state_primary] -> Selector47/1
  [z_state] -> Selector48/1
  Selector47/1 -> Mux/1
  Selector48/1 -> Mux/2
  Mux/1 -> Square1/1
  Sqrt1/1 -> Virtual Stance Leg Lengths/1
  Sqrt2/1 -> Virtual Stance Leg Lengths/2
  Mux4/1 -> Square2/1
  Selector49/1 -> Mux4/2
  [z_state] -> Selector49/1
  Square2/1 -> Sum of Elements2/1
  Sum of Elements2/1 -> Sqrt2/1
  [x_state_secondary] -> Selector46/1
  Selector46/1 -> Mux4/1
  [time_to_takeoff] -> Contact State Machine/6(Time Untill Primary Takeoff)
  [right_is_primary] -> Contact State Machine/7(Right is Primary?)
  [z_state] -> Selector50/1
  [com_velocity] -> Square3/1
  Selector50/1 -> Gain9/1
  Square3/1 -> Gain10/1
  Gain10/1 -> Gain11/1
  Gain11/1 -> Selector51/1
  Gain9/1 -> Gain13/1
  Gain13/1 -> Mux5/1
  Mux5/1 -> Energy/1, Discrete Derivative/1
  Discrete Derivative/1 -> Energy/2
  Selector42/1 -> Horizontal Force/1
  Selector43/1 -> Horizontal Force/2
  Selector44/1 -> Vertical Force/1
  Selector52/1 -> Vertical Force/2
  Selector51/1 -> Mux5/2
  [takeoff_leg] -> Contact State Machine/8(Takeoff Leg [1/2])
  [section_number] -> Section Number/1
  [right_stance] -> Detect Decrease2/1
  [left_stance] -> Detect Decrease4/1
  Detect Decrease2/1 -> Data Type Conversion/1
  Unit Delay1/1 -> Sum/2
  Sum/1 -> Unit Delay1/1, Step Count (Right/Left/Total)/1, Sum2/1
  Sum1/1 -> Unit Delay2/1, Sum2/2, Step Count (Right/Left/Total)/2
  Unit Delay2/1 -> Sum1/2
  Detect Decrease4/1 -> Data Type Conversion1/1
  Data Type Conversion/1 -> Sum/1
  Data Type Conversion1/1 -> Sum1/1
  Sum2/1 -> [step_count]
  [step_count] -> Step Count (Right/Left/Total)/3
  [double_support] -> Logical Operator10/3
  Logical Operator10/1 -> [at_rest]
  From258/1 -> Select Gait Number/1(system_time)
  From259/1 -> Select Gait Number/2(step_number)
  Constant4/1 -> [gait_id]
  From260/1 -> Unit Delay4/1
  Select Gait Number/2(enable_locomotion) -> Logical Operator15/1
  Select Gait Number/3(disable_locomotion) -> Logical Operator15/2
  Unit Delay4/1 -> Select Gait Number/3(at_rest)
  Mux28/1 -> Product4/2
  [motor_velocity_left] -> Mux28/2
  [motor_velocity_right] -> Mux28/1
  Logical Operator9/1 -> Product4/1
  Product4/1 -> Velocity Commands [rad/s x4]/1
  Filter Gyro Velocities/1(filtered dq) -> [dq], Select State Variables/2(dq/dt)
  [system_time] -> Sum4/2, Hold Value/1(In)
  Hold Value/1(Out) -> Sum4/1
  Logical Operator2/1 -> Hold Value/Enable
  [step_count] -> Compare To Zero/1
  Compare To Zero/1 -> Logical Operator2/1
  Detect Decrease/1 -> Logical Operator2/2
  Sum4/1 -> [time_after_first_touchdown]
  [time_after_first_touchdown] -> Compare To Constant/1
  Logical Operator6/1 -> Latch2/Enable
  [flight] -> Logical Operator6/1
  Compare To Constant/1 -> Logical Operator8/1
  Latch2/1(latched) -> Logical Operator8/2
  [controller_enabled] -> Contact State Machine/Enable
  Constant/1 -> [joint_torque_primary_swing]
  Constant5/1 -> [joint_torque_secondary_swing]
  Mux29/1 -> Motion Planner/11(Primary Foot2Com Position)
  Motion Planner/6(Time of Double Support [s]) -> [double_support_time]
  Motion Planner/14("Desired [y, dy/dt, ddy/ddt] Secondary") -> [desired_swing_y_secondary]
  [torso_pitch] -> Planar Inverse Dynamics/4(Torso Pitch [rad rad/s])
  [leg_length_secondary] -> Planar Inverse Dynamics/10(Leg Length Secondary [m m/s])
  Planar Inverse Dynamics/2("[tau_back, tau_front] Secondary") -> [joint_torque_secondary_stance]
  Selector57/1 -> Mux29/1
  [foot2com_z_primary] -> Selector58/1
  Centroidal Model Control/3(Desired X state) -> [desired_stance_state_x]
  [enable_locomotion] -> Motion Planner/10(Enable Locomotion [1/0])
  [x_state_secondary] -> Centroidal Model Control/6("[x, dx/dt] Secondary")
  2D Lateral Stance Control2/1(lateral_torque) -> [lateral_torque_secondary_stance]
  Motion Planner/15("Desired [z, dz/dt, ddz/ddt] Secondary") -> [desired_swing_z_secondary]
  [com_velocity] -> Planar Inverse Dynamics/5("[dx/dt, dz/dt]")
  Centroidal Model Control/1("Desired [Fx, Fz] Primary") -> [desired_force_primary], Planar Inverse Dynamics/2("[Fx, Fz] Primary Desired")
  [foot2com_x_primary] -> Selector57/1
  [phase] -> Centroidal Model Control/4(Phase [0/1/2])
  [axial_force_secondary] -> Selector56/1
  [x_state_primary] -> Motion Planner/4("[x, dx/dt] Primary")
  [right_is_primary] -> Motion Planner/16(Right Is Primary [1/0])
  Motion Planner/2(Stance Feedback Matrix) -> [stance_feedback]
  [torso_pitch] -> Centroidal Model Control/8(Torso Pitch [rad rad/s])
  [grf_xz_secondary] -> Motion Planner/9("[GRFx, GRFz] Secondary")
  [foot2com_z_secondary] -> Motion Planner/15("foot2com [z, dz/dt] secondary")
  Centroidal Model Control/4(Desired Z state) -> [desired_stance_state_z]
  Motion Planner/5(To Double Support [true/false]) -> [touchdown_will_occur]
  [leg_angle_secondary] -> Planar Inverse Dynamics/9(Leg Angle Secondary [rad rad/s])
  Selector56/1 -> 2D Lateral Stance Control2/1(F_leg)
  Motion Planner/10("Desired [x, dx/dt, ddx/ddt] Primary") -> [desired_swing_x_primary]
  Motion Planner/12("Desired [z, dz/dt, ddz/ddt] Primary") -> [desired_swing_z_primary]
  [system_time] -> Motion Planner/2(System Time [s])
  Motion Planner/3(Stance Feedforward) -> [stance_feedforward]
  Selector58/1 -> Mux29/2
  [z_state] -> Motion Planner/6("[z, dz/dt]")
  [x_state_secondary] -> Motion Planner/5("[x, dx/dt] Secondary")
  [foot2com_x_secondary] -> Motion Planner/14("foot2com [x, dx/dt] secondary")
  [foot2com_z_primary] -> Motion Planner/13("foot2com [z, dz/dt] primary")
  Motion Planner/11("Desired [y, dy/dt, ddy/ddt] Primary") -> [desired_swing_y_primary]
  [phase] -> Motion Planner/3(Phase [0/1/2])
  [leg_angle_primary] -> Planar Inverse Dynamics/6(Leg Angle Primary [rad rad/s])
  [stance_feedback] -> Centroidal Model Control/2(Feedback Matrix)
  [stance_feedforward] -> Centroidal Model Control/3(Feedforward Terms)
  [leg_length_primary] -> Planar Inverse Dynamics/7(Leg Length Primary [m m/s])
  [leg_length_secondary] -> Centroidal Model Control/10(Leg Length Secondary)
  Motion Planner/7(TIme Until Primary Takeoff [s]) -> [time_to_takeoff]
  [com_accel_z] -> Centroidal Model Control/11(CoM Acceleration Z)
  [x_state_primary] -> Centroidal Model Control/5("[x, dx/dt] Primary")
  [leg_width_secondary] -> Planar Inverse Dynamics/11(Leg Width Secondary [m m/s])
  [stance_reference] -> Centroidal Model Control/1(State Reference)
  Motion Planner/1(Stance State Reference) -> [stance_reference]
  Motion Planner/13("Desired [x, dx/dt, ddx/ddt] Secondary") -> [desired_swing_x_secondary]
  Planar Inverse Dynamics/1("[tau_back, tau_front] Primary") -> [joint_torque_primary_stance]
  [pelvis2com_pos] -> Planar Inverse Dynamics/12(Pelvis to CoM Position)
  [leg_length_primary] -> Centroidal Model Control/9(Leg Length Primary)
  [foot2com_x_primary] -> Motion Planner/12("foot2com [x, dx/dt] primary")
  Selector55/1 -> 2D Lateral Stance Control3/1(F_leg)
  Motion Planner/4(Angle of Attack [deg]) -> [angle_of_attack]
  [z_state] -> Centroidal Model Control/7("[z, dz/dt]")
  [axial_force_primary] -> Selector55/1
  Motion Planner/8(Takeoff Leg Number [1/2]) -> [takeoff_leg]
  [phase] -> Planar Inverse Dynamics/1(Phase [0/1/2])
  [grf_xz_secondary] -> Centroidal Model Control/13("[GRFx, GRFz] Secondary")
  Centroidal Model Control/2("Desired [Fx, Fz] Secondary") -> [desired_force_secondary], Planar Inverse Dynamics/3("[Fx, Fz] Secondary Desired")
  [leg_width_primary] -> Planar Inverse Dynamics/8(Leg Width Primary [m m/s])
  [torso_pitch] -> Motion Planner/7("Torso Pitch [rad, rad/s]")
  [enable_locomotion] -> Centroidal Model Control/14(Enable Locomotion [true/false])
  [grf_xz_primary] -> Centroidal Model Control/12("[GRFx, GRFz] Primary")
  Motion Planner/9(Section Number [1/2/3]) -> [section_number]
  [gait_id] -> Motion Planner/1(Gait ID [1/2/3])
  2D Lateral Stance Control3/1(lateral_torque) -> [lateral_torque_primary_stance]
  [grf_xz_primary] -> Motion Planner/8("[GRFx, GRFz] Primary")
  Mux8/1 -> Filter Torques/1(in)
  Filter Torques/1(out) -> SEA Torque Commands [Nm] x4/1
  [right_is_primary] -> Centroidal Model Control/15(Right is Primary [true/false])
  Motion Planner/16(Plan Not Ready [true/false]) -> [plan_not_ready]
  [plan_not_ready] -> Centroidal Model Control/16(Plan Not Ready [true/false])
  [plan_not_ready] -> Swing Leg Control Primary/15(Plan Not Ready [true/false])
  [plan_not_ready] -> Swing Leg Control Secondary/15(Plan Not Ready [true/false])
  [plan_not_ready] -> Plan Not Ready/1

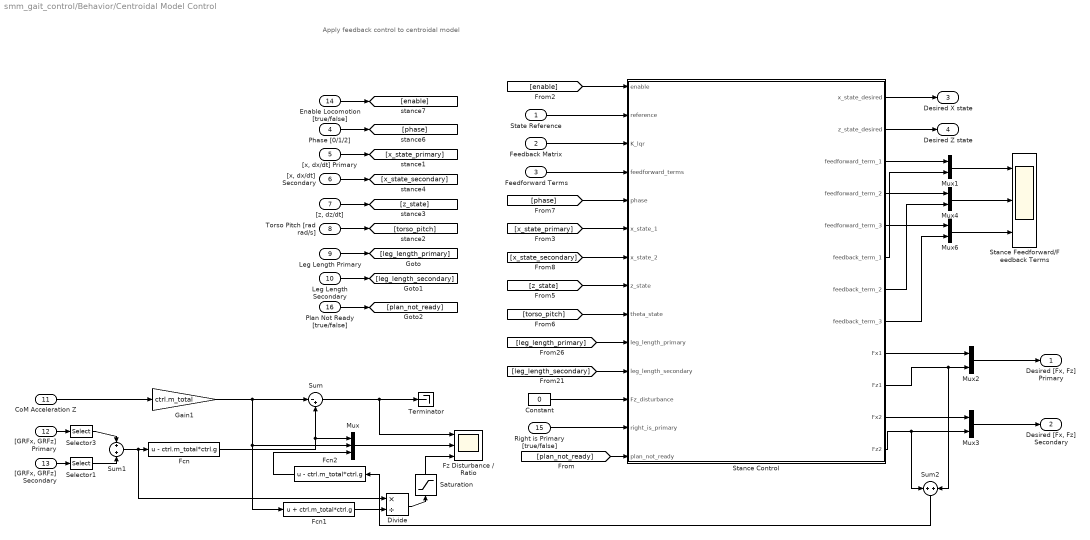
== system smm_gait_control/Behavior/Centroidal Model Control ==
  note: Apply feedback control to centroidal model
  State Reference : Inport
  Feedback Matrix : Inport  Port=2
  Feedforward Terms : Inport  Port=3
  Phase [0/1/2] : Inport  Port=4
  "[x, dx/dt] Primary" : Inport  Port=5
  "[x, dx/dt] Secondary" : Inport  Port=6
  "[z, dz/dt]" : Inport  Port=7
  Torso Pitch [rad rad/s] : Inport  Port=8
  Leg Length Primary : Inport  Port=9
  Leg Length Secondary : Inport  Port=10
  CoM Acceleration Z : Inport  Port=11
  "[GRFx, GRFz] Primary" : Inport  Port=12
  "[GRFx, GRFz] Secondary" : Inport  Port=13
  Enable Locomotion [true/false] : Inport  Port=14
  Right is Primary [true/false] : Inport  Port=15
  Plan Not Ready [true/false] : Inport  Port=16
  Constant : Constant  Value=0
  Divide : Product  Inputs=*/
  Fcn : Fcn  Expr=u - ctrl.m_total*ctrl.g
  Fcn1 : Fcn  Expr=u + ctrl.m_total*ctrl.g
  Fcn2 : Fcn  Expr=u - ctrl.m_total*ctrl.g
  Fz Disturbance / Ratio : Scope  NumInputPorts=3
  Gain1 : Gain  Gain=ctrl.m_total
  Mux : Mux  Inputs=3
  Mux{1..4,6} (5 alike) : Mux  Inputs=2
  Saturation : Saturate  UpperLimit=1.5  LowerLimit=0.5
  Selector1 : Selector  InputPortWidth=2  IndexOptions=Index vector (dialog)  Indices=[2]  OutputSizes=1
  Selector3 : Selector  InputPortWidth=2  IndexOptions=Index vector (dialog)  Indices=[2]  OutputSizes=1
  Stance Control : MATLAB Function  TreatAsAtomicUnit=on
  Stance Feedforward/Feedback Terms : Scope  NumInputPorts=3
  Sum : Sum  Inputs=|-+
  Sum1 : Sum  Inputs=+|+
  Sum2 : Sum
  Terminator : Terminator
  "Desired [Fx, Fz] Primary" : Outport
  "Desired [Fx, Fz] Secondary" : Outport  Port=2
  Desired X state : Outport  Port=3
  Desired Z state : Outport  Port=4
  wires:
  Mux2/1 -> "Desired [Fx, Fz] Primary"/1
  "[z, dz/dt]"/1 -> [z_state]
  "[x, dx/dt] Primary"/1 -> [x_state_primary]
  Torso Pitch [rad rad/s]/1 -> [torso_pitch]
  "[x, dx/dt] Secondary"/1 -> [x_state_secondary]
  Phase [0/1/2]/1 -> [phase]
  Mux3/1 -> "Desired [Fx, Fz] Secondary"/1
  Stance Control/9(Fx1) -> Mux2/1
  Stance Control/10(Fz1) -> Sum2/2, Mux2/2
  Stance Control/11(Fx2) -> Mux3/1
  Stance Control/12(Fz2) -> Mux3/2, Sum2/1
  Enable Locomotion [true/false]/1 -> [enable]
  Stance Control/1(x_state_desired) -> Desired X state/1
  Stance Control/2(z_state_desired) -> Desired Z state/1
  Mux1/1 -> Stance Feedforward/Feedback Terms/1
  Stance Control/3(feedforward_term_1) -> Mux1/1
  Stance Control/6(feedback_term_1) -> Mux1/2
  Mux4/1 -> Stance Feedforward/Feedback Terms/2
  Mux6/1 -> Stance Feedforward/Feedback Terms/3
  Stance Control/4(feedforward_term_2) -> Mux4/1
  Stance Control/7(feedback_term_2) -> Mux4/2
  Stance Control/5(feedforward_term_3) -> Mux6/1
  Stance Control/8(feedback_term_3) -> Mux6/2
  Leg Length Secondary/1 -> [leg_length_secondary]
  Leg Length Primary/1 -> [leg_length_primary]
  [enable] -> Stance Control/1(enable)
  [leg_length_secondary] -> Stance Control/11(leg_length_secondary)
  [leg_length_primary] -> Stance Control/10(leg_length_primary)
  [torso_pitch] -> Stance Control/9(theta_state)
  [z_state] -> Stance Control/8(z_state)
  [x_state_secondary] -> Stance Control/7(x_state_2)
  [x_state_primary] -> Stance Control/6(x_state_1)
  [phase] -> Stance Control/5(phase)
  State Reference/1 -> Stance Control/2(reference)
  Feedback Matrix/1 -> Stance Control/3(K_lqr)
  Feedforward Terms/1 -> Stance Control/4(feedforward_terms)
  Selector3/1 -> Sum1/1
  "[GRFx, GRFz] Secondary"/1 -> Selector1/1
  Selector1/1 -> Sum1/2
  Sum1/1 -> Divide/1, Fcn/1
  Fcn/1 -> Mux/1, Sum/2
  CoM Acceleration Z/1 -> Gain1/1
  Gain1/1 -> Mux/2, Fcn1/1, Sum/1
  "[GRFx, GRFz] Primary"/1 -> Selector3/1
  Sum/1 -> Terminator/1, Fz Disturbance / Ratio/1
  Divide/1 -> Saturation/1
  Mux/1 -> Fz Disturbance / Ratio/2
  Fcn1/1 -> Divide/2
  Fcn2/1 -> Mux/3
  Right is Primary [true/false]/1 -> Stance Control/13(right_is_primary)
  Constant/1 -> Stance Control/12(Fz_disturbance)
  Plan Not Ready [true/false]/1 -> [plan_not_ready]
  [plan_not_ready] -> Stance Control/14(plan_not_ready)
  Saturation/1 -> Fz Disturbance / Ratio/3
  Sum2/1 -> Fcn2/1

== system smm_gait_control/Behavior/CoM Kinematics ==
  Torso Roll : Inport
  Torso Pitch : Inport  Port=2
  Torso Yaw : Inport  Port=3
  Leg Angle Right : Inport  Port=4
  Leg Roll Right : Inport  Port=5
  Leg Length Right : Inport  Port=6
  Leg Angle Left : Inport  Port=7
  Leg Roll Left : Inport  Port=8
  Leg Length Left : Inport  Port=9
  Mux{,1..3} (4 alike) : Mux  Inputs=2
  PositionUsingRobotGeometry : MATLAB Function  TreatAsAtomicUnit=on
  Selector{,1,4..5} (4 alike) : Selector  InputPortWidth=3  IndexOptions=Index vector (dialog)  Indices=[1]  OutputSizes=1
  Selector{2..3,6..7} (4 alike) : Selector  InputPortWidth=3  IndexOptions=Index vector (dialog)  Indices=[3]  OutputSizes=1
  Terminator{,1..3} (4 alike) : Terminator
  Foot2CoM Pos Left Yawed [m] x3 : Outport
  Foot2CoM Vel Left Yawed [m/s] x3 : Outport  Port=2
  Foot2CoM Pos Right Yawed [m] x3 : Outport  Port=3
  Foot2CoM Vel Right Yawed [m/s] x3 : Outport  Port=4
  Pelvis2CoM Pos Body [m] x3 : Outport  Port=5
  Pelvis2CoM Vel Body [m/s] x3 : Outport  Port=6
  Foot2CoM X State Left [m m/s] : Outport  Port=7
  Foot2CoM Z State Left [m m/s] : Outport  Port=8
  Foot2CoM X State Right [m m/s] : Outport  Port=9
  Foot2CoM Z State Right [m m/s] : Outport  Port=10
  wires:
  Leg Angle Left/1 -> PositionUsingRobotGeometry/4(left_leg_sagittal_angle)
  Leg Roll Left/1 -> PositionUsingRobotGeometry/5(left_leg_lateral_angle)
  Leg Length Left/1 -> PositionUsingRobotGeometry/6(left_leg_length)
  Leg Angle Right/1 -> PositionUsingRobotGeometry/7(right_leg_sagittal_angle)
  Leg Roll Right/1 -> PositionUsingRobotGeometry/8(right_leg_lateral_angle)
  Leg Length Right/1 -> PositionUsingRobotGeometry/9(right_leg_length)
  Torso Roll/1 -> PositionUsingRobotGeometry/1(roll)
  Torso Yaw/1 -> PositionUsingRobotGeometry/3(yaw)
  Torso Pitch/1 -> PositionUsingRobotGeometry/2(pitch)
  PositionUsingRobotGeometry/3(com_right_yawed) -> Selector4/1, Selector6/1, Foot2CoM Pos Right Yawed [m] x3/1
  PositionUsingRobotGeometry/4(dcom_right_yawed) -> Selector5/1, Selector7/1, Foot2CoM Vel Right Yawed [m/s] x3/1
  PositionUsingRobotGeometry/1(com_left_yawed) -> Foot2CoM Pos Left Yawed [m] x3/1, Selector2/1, Selector/1
  PositionUsingRobotGeometry/2(dcom_left_yawed) -> Selector3/1, Foot2CoM Vel Left Yawed [m/s] x3/1, Selector1/1
  PositionUsingRobotGeometry/10(dcom_pelvis_body) -> Pelvis2CoM Vel Body [m/s] x3/1
  PositionUsingRobotGeometry/9(com_pelvis_body) -> Pelvis2CoM Pos Body [m] x3/1
  PositionUsingRobotGeometry/5(com_left_global) -> Terminator/1
  PositionUsingRobotGeometry/6(dcom_left_global) -> Terminator1/1
  PositionUsingRobotGeometry/7(com_right_global) -> Terminator2/1
  PositionUsingRobotGeometry/8(dcom_right_global) -> Terminator3/1
  Selector/1 -> Mux/1
  Selector1/1 -> Mux/2
  Mux/1 -> Foot2CoM X State Left [m m/s]/1
  Selector3/1 -> Mux1/2
  Selector2/1 -> Mux1/1
  Mux1/1 -> Foot2CoM Z State Left [m m/s]/1
  Mux3/1 -> Foot2CoM Z State Right [m m/s]/1
  Selector6/1 -> Mux3/1
  Selector7/1 -> Mux3/2
  Mux2/1 -> Foot2CoM X State Right [m m/s]/1
  Selector5/1 -> Mux2/2
  Selector4/1 -> Mux2/1
